simulink model "electric_motor_and_propeller"  (R2022a)
settings: Solver=ode1  StartTime=0.0  StopTime=20  FixedStep=0.01  RelTol=1e-3
values from neighbouring files (symbols this model uses):
  motor =     [electric_motor_and_propeller.mat]
  propeller =     [electric_motor_and_propeller.mat]
settings Model: Creator=kboychev  LastModifiedBy=Kiril Boychev
settings SolverCC: AlgebraicLoopSolver=TrustRegion
settings DataIOCC: ReturnWorkspaceOutputs=off
settings DebuggingCC: UnconnectedInputMsg=warning  UnconnectedOutputMsg=warning  UnconnectedLineMsg=warning  SFMachineParentedDataDiag=warning  ArithmeticOperatorsInVariantConditions=warning
settings SFSimCC: CustomCodeUndefinedFunction=UseInterfaceOnly

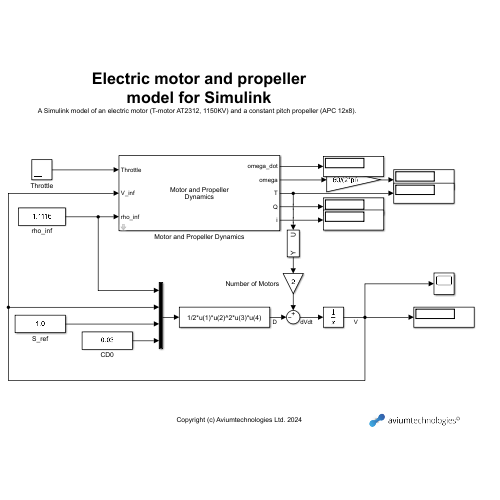
[thumbnail: Simulink's stored preview of the top-level diagram]
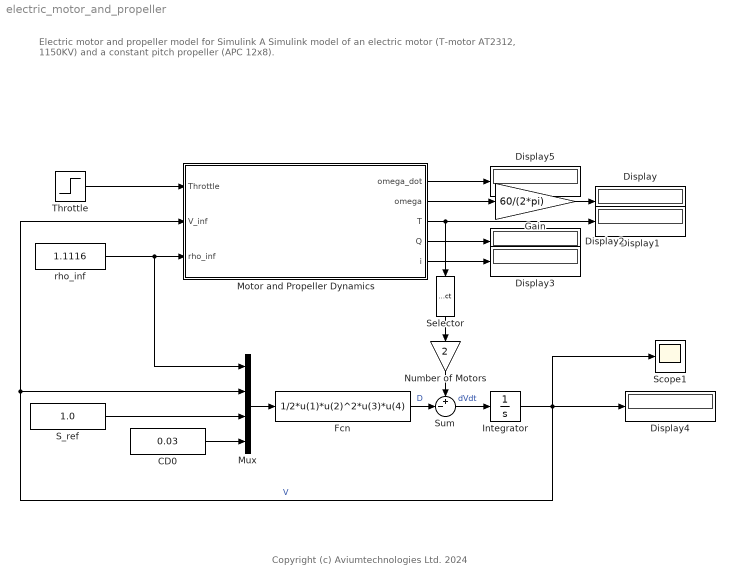
== system electric_motor_and_propeller ==
  note: Copyright (c) Aviumtechnologies Ltd. 2024
  note: Electric motor and propeller
      | model for Simulink
      | A Simulink model of an electric motor (T-motor AT2312, 1150KV) and a constant pitch propeller (APC 12x8).
  CD0 : Constant  Value=0.03
  Display{,1..5} (6 alike) : Display
  Fcn : Fcn  Expr=1/2*u(1)*u(2)^2*u(3)*u(4)
  Gain : Gain  Gain=60/(2*pi)
  Integrator : Integrator
  Motor and Propeller Dynamics : Subsystem  mask(Electric motor and fixed-pitch propeller dynamics){i0=motor.i0, omega0=motor.omega0, max_voltage=motor.max_voltage, Kv=motor.Kv, R=motor.R, L=motor.H, axis_of_rotation=motor.axis_of_rotation, direction_of_rotation=motor.direction_of_rotation, J=propeller.J, D=propeller.D, CT_lookup=propeller.CT_lookup, CP_lookup=propeller.CP_lookup, J_lookup=propeller.J_lookup, omega_lookup=propeller.omega_lookup}
      mask prompts: i0 "Initial motor current (A)"; omega0 "Initial motor speed (rad/s)"; max_voltage "Motor maximum voltage (V)"; Kv "Motor speed constant (rad/s/V)"; R "Motor resistance (Ohm)"; L "Motor inductance (H)"; axis_of_rotation "Motor axis of rotation (-)"; direction_of_rotation "Motor direction of rotation (-)"; J "Propeller moment of inertia (kg.m^2)"; D "Propeller diamater (m)"; CT_lookup "Propeller thrust coefficient 2D lookup table"; CP_lookup "Propeller power coefficient 2D lookup table"; J_lookup "Propeller advance ratio lookup vector"; omega_lookup "Propeller speed lookup vector"
      mask help: Electric motor and fixed-pitch propeller dynamics using look-up tables of thrust and power coefficients as functions of advance ratio and rotation speed.The electric model is modelled by two first-order differential equations - one for the current and one for the rotational speed.
      mask DialogControl Container5 Prompt: Main
      mask Display: fprintf('Motor and Propeller\nDynamics');
  Mux : Mux
  Number of Motors : Gain  Gain=2
  S_ref : Constant  Value=1.0
  Scope1 : Scope
  Selector : Selector  IndexMode=Zero-based  InputPortWidth=3  IndexOptions=Index vector (dialog)  Indices=0  OutputSizes=1
  Sum : Sum  Inputs=+-|
  Throttle : Step  SampleTime=0
  rho_inf : Constant  Value=1.1116
  wires:
  Integrator/1 -> Display4/1, Scope1/1, Motor and Propeller Dynamics/2(V_inf), Mux/2  "V"
  Motor and Propeller Dynamics/2(omega) -> Gain/1
  Motor and Propeller Dynamics/3(T) -> Display1/1, Selector/1
  Motor and Propeller Dynamics/4(Q) -> Display2/1
  Motor and Propeller Dynamics/5(i) -> Display3/1
  Gain/1 -> Display/1
  Fcn/1 -> Sum/2  "D"
  Sum/1 -> Integrator/1  "dVdt"
  Mux/1 -> Fcn/1
  S_ref/1 -> Mux/3
  CD0/1 -> Mux/4
  Throttle/1 -> Motor and Propeller Dynamics/1(Throttle)
  Selector/1 -> Number of Motors/1
  Motor and Propeller Dynamics/1(omega_dot) -> Display5/1
  Number of Motors/1 -> Sum/1
  rho_inf/1 -> Motor and Propeller Dynamics/3(rho_inf), Mux/1

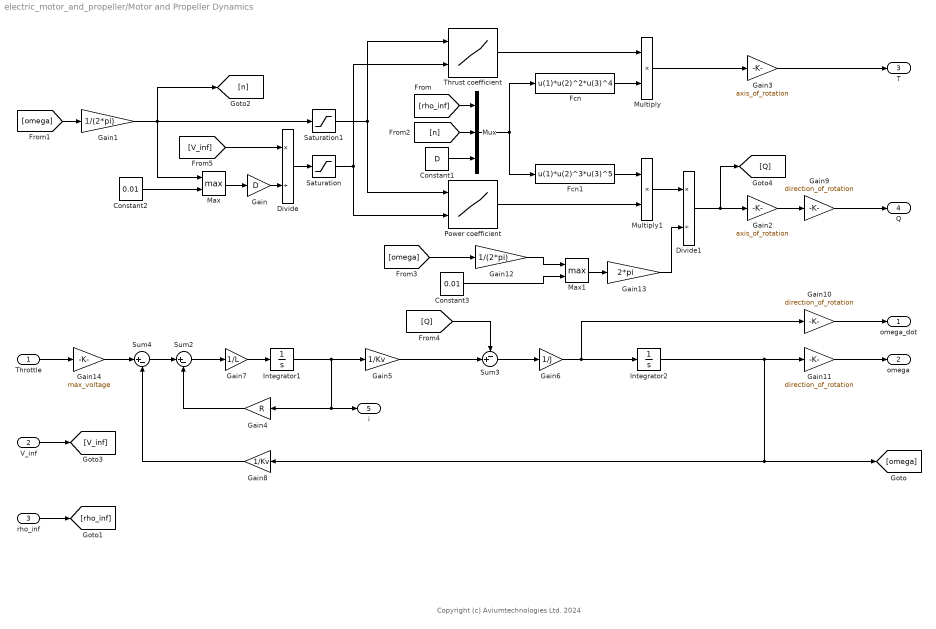
== system electric_motor_and_propeller/Motor and Propeller Dynamics ==
  note: Copyright (c) Aviumtechnologies Ltd. 2024
  Throttle : Inport
  V_inf : Inport  Port=2
  rho_inf : Inport  Port=3
  Constant1 : Constant  Value=D
  Constant2 : Constant  Value=0.01
  Constant3 : Constant  Value=0.01
  Divide : Product  Inputs=*/
  Divide1 : Product  Inputs=*/
  Fcn : Fcn  Expr=u(1)*u(2)^2*u(3)^4
  Fcn1 : Fcn  Expr=u(1)*u(2)^3*u(3)^5
  Gain : Gain  Gain=D
  Gain1 : Gain  Gain=1/(2*pi)
  Gain10 : Gain  Gain=direction_of_rotation
  Gain11 : Gain  Gain=direction_of_rotation
  Gain12 : Gain  Gain=1/(2*pi)
  Gain13 : Gain  Gain=2*pi
  Gain14 : Gain  Gain=max_voltage
  Gain2 : Gain  Gain=axis_of_rotation
  Gain3 : Gain  Gain=axis_of_rotation
  Gain4 : Gain  Gain=R
  Gain5 : Gain  Gain=1/Kv
  Gain6 : Gain  Gain=1/J
  Gain7 : Gain  Gain=1/L
  Gain8 : Gain  Gain=1/Kv
  Gain9 : Gain  Gain=direction_of_rotation
  Integrator1 : Integrator  InitialCondition=i0
  Integrator2 : Integrator  InitialCondition=omega0
  Max : MinMax  Function=max  Inputs=2
  Max1 : MinMax  Function=max  Inputs=2
  Multiply : Product
  Multiply1 : Product
  Mux : Mux  Inputs=3
  Power coefficient : Lookup_n-D  BreakpointsForDimension1=omega_lookup  BreakpointsForDimension2=J_lookup  Table=CP_lookup  DiagnosticForOutOfRangeInput=Warning  InternalRulePriority=Speed  RndMeth=Simplest
      settings: InputPortMap=u0,u1
  Saturation : Saturate  UpperLimit=max(J_lookup)  LowerLimit=min(J_lookup)
  Saturation1 : Saturate  UpperLimit=max(omega_lookup)  LowerLimit=min(omega_lookup)
  Sum2 : Sum  Inputs=|+-
  Sum3 : Sum  Inputs=-+|
  Sum4 : Sum  Inputs=|+-
  Thrust coefficient : Lookup_n-D  BreakpointsForDimension1=omega_lookup  BreakpointsForDimension2=J_lookup  Table=CT_lookup  DiagnosticForOutOfRangeInput=Warning  InternalRulePriority=Speed  RndMeth=Simplest
      settings: InputPortMap=u0,u1
  omega_dot : Outport  VectorParamsAs1DForOutWhenUnconnected=off
  omega : Outport  Port=2  VectorParamsAs1DForOutWhenUnconnected=off
  T : Outport  Port=3  VectorParamsAs1DForOutWhenUnconnected=off
  Q : Outport  Port=4  VectorParamsAs1DForOutWhenUnconnected=off
  i : Outport  Port=5  VectorParamsAs1DForOutWhenUnconnected=off
  wires:
  Gain5/1 -> Sum3/2
  Gain8/1 -> Sum4/2
  Gain6/1 -> Gain10/1, Integrator2/1
  Sum4/1 -> Sum2/1
  Gain7/1 -> Integrator1/1
  Sum3/1 -> Gain6/1
  Gain4/1 -> Sum2/2
  Sum2/1 -> Gain7/1
  Integrator1/1 -> Gain5/1, i/1, Gain4/1
  Throttle/1 -> Gain14/1
  rho_inf/1 -> [rho_inf]
  V_inf/1 -> [V_inf]
  [omega] -> Gain1/1
  Gain1/1 -> Max/1, [n], Saturation1/1
  [V_inf] -> Divide/1
  Divide/1 -> Saturation/1
  Thrust coefficient/1 -> Multiply/1
  Power coefficient/1 -> Multiply1/2
  Fcn/1 -> Multiply/2
  [rho_inf] -> Mux/1
  [n] -> Mux/2
  Constant1/1 -> Mux/3
  Mux/1 -> Fcn/1, Fcn1/1
  Fcn1/1 -> Multiply1/1
  Multiply1/1 -> Divide1/1
  Gain/1 -> Divide/2
  Max/1 -> Gain/1
  Max1/1 -> Gain13/1
  [omega] -> Gain12/1
  Saturation/1 -> Power coefficient/2, Thrust coefficient/2
  Saturation1/1 -> Power coefficient/1, Thrust coefficient/1
  Multiply/1 -> Gain3/1
  Divide1/1 -> [Q], Gain2/1
  Integrator2/1 -> Gain11/1, Gain8/1, [omega]
  Gain9/1 -> Q/1
  Gain3/1 -> T/1
  Gain10/1 -> omega_dot/1
  Gain11/1 -> omega/1
  Constant2/1 -> Max/2
  Gain12/1 -> Max1/1
  Constant3/1 -> Max1/2
  [Q] -> Sum3/1
  Gain13/1 -> Divide1/2
  Gain2/1 -> Gain9/1
  Gain14/1 -> Sum4/1
